simulink model "model (1)"  (R2014b)
settings: Solver=ode45  StartTime=0.0  StopTime=300  RelTol=1e-3
settings Model: Creator=User  LastModifiedBy=User

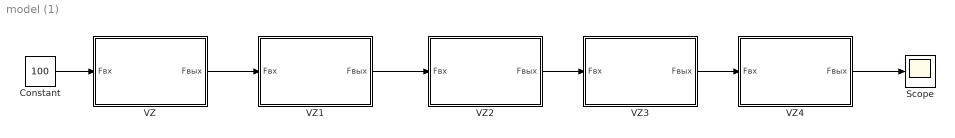
== system model (1) ==
  Constant : Constant  Value=100
  Scope : Scope
  VZ : Subsystem
  VZ1 : Subsystem
  VZ2 : Subsystem
  VZ3 : Subsystem
  VZ4 : Subsystem
  wires:
  VZ/1(Fвых) -> VZ1/1(Fвх)
  VZ4/1(Fвых) -> Scope/1
  Constant/1 -> VZ/1(Fвх)
  VZ1/1(Fвых) -> VZ2/1(Fвх)
  VZ2/1(Fвых) -> VZ3/1(Fвх)
  VZ3/1(Fвых) -> VZ4/1(Fвх)

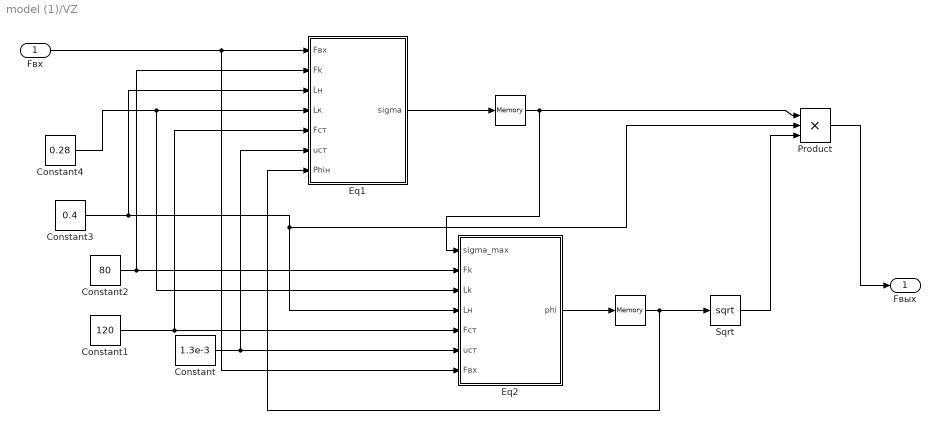
== system model (1)/VZ ==
  Fвх : Inport
  " " : Memory
  "  " : Memory
  Constant : Constant  Value=1.3e-3
  Constant1 : Constant  Value=120
  Constant2 : Constant  Value=80
  Constant3 : Constant  Value=0.4
  Constant4 : Constant  Value=0.28
  Eq1 : Subsystem  TreatAsAtomicUnit=on
  Eq2 : Subsystem  TreatAsAtomicUnit=on
  Product : Product  Inputs=3
  Sqrt : Sqrt  SaturateOnIntegerOverflow=on
  Fвых : Outport
  wires:
  Constant2/1 -> Eq2/2(Fk), Eq1/2(Fk)
  Fвх/1 -> Eq2/7(Fвх), Eq1/1(Fвх)
  Constant1/1 -> Eq1/5(Fст), Eq2/5(Fст)
  Constant4/1 -> Eq2/3(Lk), Eq1/4(Lк)
  Constant3/1 -> Eq1/3(Lн), Product/2, Eq2/4(Lн)
  Eq1/1(sigma) -> " "/1
  "  "/1 -> Eq1/7(Phiн), Sqrt/1
  " "/1 -> Product/1, Eq2/1(sigma_max)
  Eq2/1(phi) -> "  "/1
  Constant/1 -> Eq1/6(uст), Eq2/6(uст)
  Product/1 -> Fвых/1
  Sqrt/1 -> Product/3

== system model (1)/VZ1 ==
  Fвх : Inport
  " " : Memory
  "  " : Memory
  Constant : Constant  Value=1.3e-3
  Constant1 : Constant  Value=120
  Constant2 : Constant  Value=80
  Constant3 : Constant  Value=0.4
  Constant4 : Constant  Value=0.28
  Eq1 : Subsystem  TreatAsAtomicUnit=on
  Eq2 : Subsystem  TreatAsAtomicUnit=on
  Product : Product  Inputs=3
  Sqrt : Sqrt  SaturateOnIntegerOverflow=on
  Fвых : Outport
  wires:
  Constant2/1 -> Eq2/2(Fk), Eq1/2(Fk)
  Fвх/1 -> Eq2/7(Fвх), Eq1/1(Fвх)
  Constant1/1 -> Eq1/5(Fст), Eq2/5(Fст)
  Constant4/1 -> Eq2/3(Lk), Eq1/4(Lк)
  Constant3/1 -> Eq1/3(Lн), Product/2, Eq2/4(Lн)
  Eq1/1(sigma) -> " "/1
  "  "/1 -> Eq1/7(Phiн), Sqrt/1
  " "/1 -> Product/1, Eq2/1(sigma_max)
  Eq2/1(phi) -> "  "/1
  Constant/1 -> Eq1/6(uст), Eq2/6(uст)
  Product/1 -> Fвых/1
  Sqrt/1 -> Product/3

== system model (1)/VZ2 ==
  Fвх : Inport
  " " : Memory
  "  " : Memory
  Constant : Constant  Value=1.3e-3
  Constant1 : Constant  Value=120
  Constant2 : Constant  Value=80
  Constant3 : Constant  Value=0.4
  Constant4 : Constant  Value=0.28
  Eq1 : Subsystem  TreatAsAtomicUnit=on
  Eq2 : Subsystem  TreatAsAtomicUnit=on
  Product : Product  Inputs=3
  Sqrt : Sqrt  SaturateOnIntegerOverflow=on
  Fвых : Outport
  wires:
  Constant2/1 -> Eq2/2(Fk), Eq1/2(Fk)
  Fвх/1 -> Eq2/7(Fвх), Eq1/1(Fвх)
  Constant1/1 -> Eq1/5(Fст), Eq2/5(Fст)
  Constant4/1 -> Eq2/3(Lk), Eq1/4(Lк)
  Constant3/1 -> Eq1/3(Lн), Product/2, Eq2/4(Lн)
  Eq1/1(sigma) -> " "/1
  "  "/1 -> Eq1/7(Phiн), Sqrt/1
  " "/1 -> Product/1, Eq2/1(sigma_max)
  Eq2/1(phi) -> "  "/1
  Constant/1 -> Eq1/6(uст), Eq2/6(uст)
  Product/1 -> Fвых/1
  Sqrt/1 -> Product/3

== system model (1)/VZ3 ==
  Fвх : Inport
  " " : Memory
  "  " : Memory
  Constant : Constant  Value=1.3e-3
  Constant1 : Constant  Value=120
  Constant2 : Constant  Value=80
  Constant3 : Constant  Value=0.4
  Constant4 : Constant  Value=0.28
  Eq1 : Subsystem  TreatAsAtomicUnit=on
  Eq2 : Subsystem  TreatAsAtomicUnit=on
  Product : Product  Inputs=3
  Sqrt : Sqrt  SaturateOnIntegerOverflow=on
  Fвых : Outport
  wires:
  Constant2/1 -> Eq2/2(Fk), Eq1/2(Fk)
  Fвх/1 -> Eq2/7(Fвх), Eq1/1(Fвх)
  Constant1/1 -> Eq1/5(Fст), Eq2/5(Fст)
  Constant4/1 -> Eq2/3(Lk), Eq1/4(Lк)
  Constant3/1 -> Eq1/3(Lн), Product/2, Eq2/4(Lн)
  Eq1/1(sigma) -> " "/1
  "  "/1 -> Eq1/7(Phiн), Sqrt/1
  " "/1 -> Product/1, Eq2/1(sigma_max)
  Eq2/1(phi) -> "  "/1
  Constant/1 -> Eq1/6(uст), Eq2/6(uст)
  Product/1 -> Fвых/1
  Sqrt/1 -> Product/3

== system model (1)/VZ4 ==
  Fвх : Inport
  " " : Memory
  "  " : Memory
  Constant : Constant  Value=1.3e-3
  Constant1 : Constant  Value=120
  Constant2 : Constant  Value=80
  Constant3 : Constant  Value=0.4
  Constant4 : Constant  Value=0.28
  Eq1 : Subsystem  TreatAsAtomicUnit=on
  Eq2 : Subsystem  TreatAsAtomicUnit=on
  Product : Product  Inputs=3
  Sqrt : Sqrt  SaturateOnIntegerOverflow=on
  Fвых : Outport
  wires:
  Constant2/1 -> Eq2/2(Fk), Eq1/2(Fk)
  Fвх/1 -> Eq2/7(Fвх), Eq1/1(Fвх)
  Constant1/1 -> Eq1/5(Fст), Eq2/5(Fст)
  Constant4/1 -> Eq2/3(Lk), Eq1/4(Lк)
  Constant3/1 -> Eq1/3(Lн), Product/2, Eq2/4(Lн)
  Eq1/1(sigma) -> " "/1
  "  "/1 -> Eq1/7(Phiн), Sqrt/1
  " "/1 -> Product/1, Eq2/1(sigma_max)
  Eq2/1(phi) -> "  "/1
  Constant/1 -> Eq1/6(uст), Eq2/6(uст)
  Product/1 -> Fвых/1
  Sqrt/1 -> Product/3

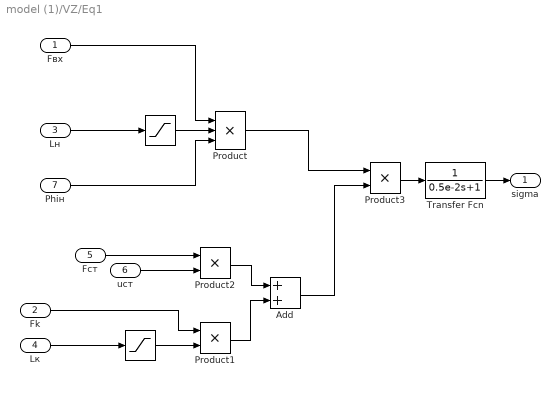
== system model (1)/VZ/Eq1 ==
  Fвх : Inport
  Fk : Inport  Port=2
  Lн : Inport  Port=3
  Lк : Inport  Port=4
  Fст : Inport  Port=5
  uст : Inport  Port=6
  Phiн : Inport  Port=7
  " " : Saturate
  "  " : Saturate
  Add : Sum
  Product : Product  Inputs=3
  Product1 : Product
  Product2 : Product
  Product3 : Product  Inputs=**
  Transfer Fcn : TransferFcn  Denominator=[0.5e-2 1]
  sigma : Outport
  wires:
  Lн/1 -> " "/1
  Lк/1 -> "  "/1
  " "/1 -> Product/2
  Fвх/1 -> Product/1
  Phiн/1 -> Product/3
  "  "/1 -> Product1/2
  Fk/1 -> Product1/1
  Fст/1 -> Product2/1
  uст/1 -> Product2/2
  Product2/1 -> Add/1
  Product1/1 -> Add/2
  Product/1 -> Product3/1
  Add/1 -> Product3/2
  Product3/1 -> Transfer Fcn/1
  Transfer Fcn/1 -> sigma/1

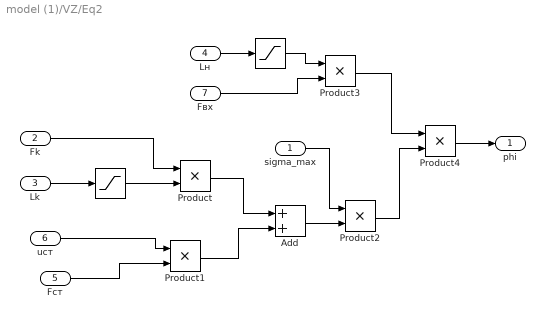
== system model (1)/VZ/Eq2 ==
  sigma_max : Inport
  Fk : Inport  Port=2
  Lk : Inport  Port=3
  Lн : Inport  Port=4
  Fст : Inport  Port=5
  uст : Inport  Port=6
  Fвх : Inport  Port=7
  " " : Saturate
  "  " : Saturate
  Add : Sum
  Product{,1..3} (4 alike) : Product
  Product4 : Product  Inputs=**
  phi : Outport
  wires:
  Lk/1 -> " "/1
  " "/1 -> Product/2
  Fk/1 -> Product/1
  uст/1 -> Product1/1
  Product/1 -> Add/1
  Product1/1 -> Add/2
  Fст/1 -> Product1/2
  Lн/1 -> "  "/1
  Add/1 -> Product2/2
  sigma_max/1 -> Product2/1
  "  "/1 -> Product3/1
  Fвх/1 -> Product3/2
  Product3/1 -> Product4/1
  Product2/1 -> Product4/2
  Product4/1 -> phi/1

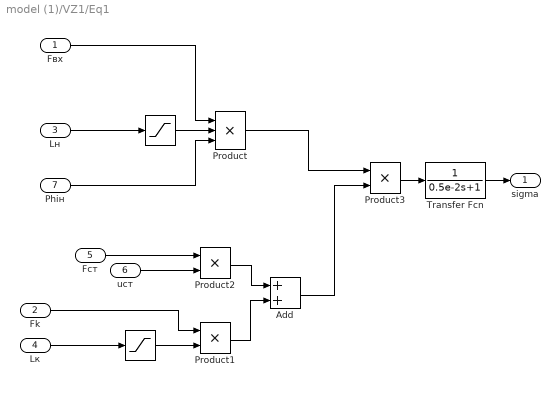
== system model (1)/VZ1/Eq1 ==
  Fвх : Inport
  Fk : Inport  Port=2
  Lн : Inport  Port=3
  Lк : Inport  Port=4
  Fст : Inport  Port=5
  uст : Inport  Port=6
  Phiн : Inport  Port=7
  " " : Saturate
  "  " : Saturate
  Add : Sum
  Product : Product  Inputs=3
  Product1 : Product
  Product2 : Product
  Product3 : Product  Inputs=**
  Transfer Fcn : TransferFcn  Denominator=[0.5e-2 1]
  sigma : Outport
  wires:
  Lн/1 -> " "/1
  Lк/1 -> "  "/1
  " "/1 -> Product/2
  Fвх/1 -> Product/1
  Phiн/1 -> Product/3
  "  "/1 -> Product1/2
  Fk/1 -> Product1/1
  Fст/1 -> Product2/1
  uст/1 -> Product2/2
  Product2/1 -> Add/1
  Product1/1 -> Add/2
  Product/1 -> Product3/1
  Add/1 -> Product3/2
  Product3/1 -> Transfer Fcn/1
  Transfer Fcn/1 -> sigma/1

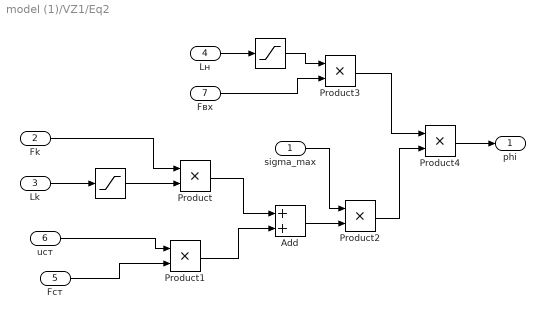
== system model (1)/VZ1/Eq2 ==
  sigma_max : Inport
  Fk : Inport  Port=2
  Lk : Inport  Port=3
  Lн : Inport  Port=4
  Fст : Inport  Port=5
  uст : Inport  Port=6
  Fвх : Inport  Port=7
  " " : Saturate
  "  " : Saturate
  Add : Sum
  Product{,1..3} (4 alike) : Product
  Product4 : Product  Inputs=**
  phi : Outport
  wires:
  Lk/1 -> " "/1
  " "/1 -> Product/2
  Fk/1 -> Product/1
  uст/1 -> Product1/1
  Product/1 -> Add/1
  Product1/1 -> Add/2
  Fст/1 -> Product1/2
  Lн/1 -> "  "/1
  Add/1 -> Product2/2
  sigma_max/1 -> Product2/1
  "  "/1 -> Product3/1
  Fвх/1 -> Product3/2
  Product3/1 -> Product4/1
  Product2/1 -> Product4/2
  Product4/1 -> phi/1

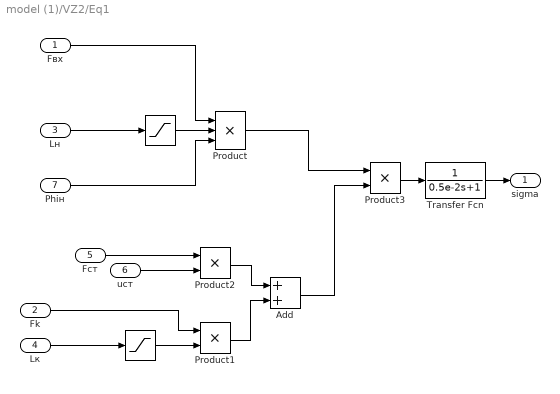
== system model (1)/VZ2/Eq1 ==
  Fвх : Inport
  Fk : Inport  Port=2
  Lн : Inport  Port=3
  Lк : Inport  Port=4
  Fст : Inport  Port=5
  uст : Inport  Port=6
  Phiн : Inport  Port=7
  " " : Saturate
  "  " : Saturate
  Add : Sum
  Product : Product  Inputs=3
  Product1 : Product
  Product2 : Product
  Product3 : Product  Inputs=**
  Transfer Fcn : TransferFcn  Denominator=[0.5e-2 1]
  sigma : Outport
  wires:
  Lн/1 -> " "/1
  Lк/1 -> "  "/1
  " "/1 -> Product/2
  Fвх/1 -> Product/1
  Phiн/1 -> Product/3
  "  "/1 -> Product1/2
  Fk/1 -> Product1/1
  Fст/1 -> Product2/1
  uст/1 -> Product2/2
  Product2/1 -> Add/1
  Product1/1 -> Add/2
  Product/1 -> Product3/1
  Add/1 -> Product3/2
  Product3/1 -> Transfer Fcn/1
  Transfer Fcn/1 -> sigma/1

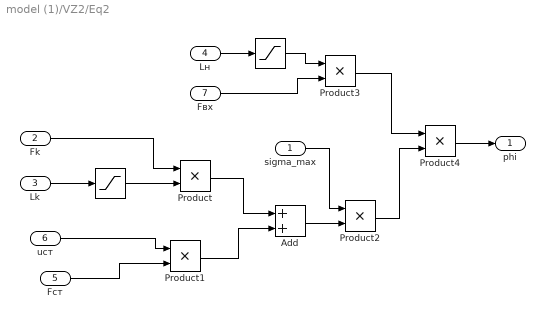
== system model (1)/VZ2/Eq2 ==
  sigma_max : Inport
  Fk : Inport  Port=2
  Lk : Inport  Port=3
  Lн : Inport  Port=4
  Fст : Inport  Port=5
  uст : Inport  Port=6
  Fвх : Inport  Port=7
  " " : Saturate
  "  " : Saturate
  Add : Sum
  Product{,1..3} (4 alike) : Product
  Product4 : Product  Inputs=**
  phi : Outport
  wires:
  Lk/1 -> " "/1
  " "/1 -> Product/2
  Fk/1 -> Product/1
  uст/1 -> Product1/1
  Product/1 -> Add/1
  Product1/1 -> Add/2
  Fст/1 -> Product1/2
  Lн/1 -> "  "/1
  Add/1 -> Product2/2
  sigma_max/1 -> Product2/1
  "  "/1 -> Product3/1
  Fвх/1 -> Product3/2
  Product3/1 -> Product4/1
  Product2/1 -> Product4/2
  Product4/1 -> phi/1

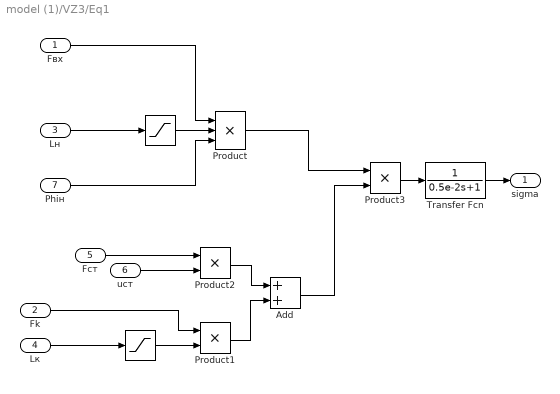
== system model (1)/VZ3/Eq1 ==
  Fвх : Inport
  Fk : Inport  Port=2
  Lн : Inport  Port=3
  Lк : Inport  Port=4
  Fст : Inport  Port=5
  uст : Inport  Port=6
  Phiн : Inport  Port=7
  " " : Saturate
  "  " : Saturate
  Add : Sum
  Product : Product  Inputs=3
  Product1 : Product
  Product2 : Product
  Product3 : Product  Inputs=**
  Transfer Fcn : TransferFcn  Denominator=[0.5e-2 1]
  sigma : Outport
  wires:
  Lн/1 -> " "/1
  Lк/1 -> "  "/1
  " "/1 -> Product/2
  Fвх/1 -> Product/1
  Phiн/1 -> Product/3
  "  "/1 -> Product1/2
  Fk/1 -> Product1/1
  Fст/1 -> Product2/1
  uст/1 -> Product2/2
  Product2/1 -> Add/1
  Product1/1 -> Add/2
  Product/1 -> Product3/1
  Add/1 -> Product3/2
  Product3/1 -> Transfer Fcn/1
  Transfer Fcn/1 -> sigma/1

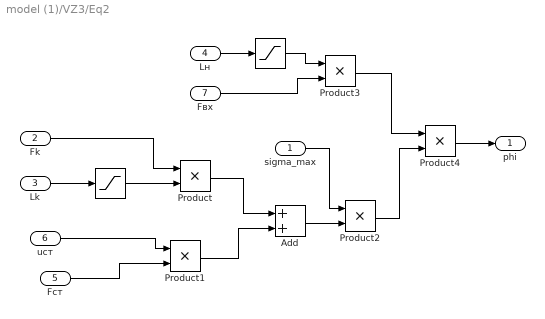
== system model (1)/VZ3/Eq2 ==
  sigma_max : Inport
  Fk : Inport  Port=2
  Lk : Inport  Port=3
  Lн : Inport  Port=4
  Fст : Inport  Port=5
  uст : Inport  Port=6
  Fвх : Inport  Port=7
  " " : Saturate
  "  " : Saturate
  Add : Sum
  Product{,1..3} (4 alike) : Product
  Product4 : Product  Inputs=**
  phi : Outport
  wires:
  Lk/1 -> " "/1
  " "/1 -> Product/2
  Fk/1 -> Product/1
  uст/1 -> Product1/1
  Product/1 -> Add/1
  Product1/1 -> Add/2
  Fст/1 -> Product1/2
  Lн/1 -> "  "/1
  Add/1 -> Product2/2
  sigma_max/1 -> Product2/1
  "  "/1 -> Product3/1
  Fвх/1 -> Product3/2
  Product3/1 -> Product4/1
  Product2/1 -> Product4/2
  Product4/1 -> phi/1

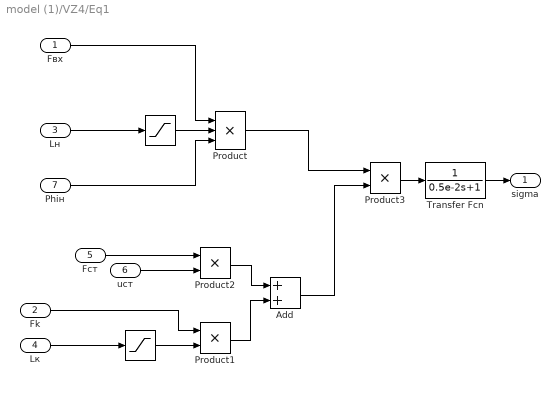
== system model (1)/VZ4/Eq1 ==
  Fвх : Inport
  Fk : Inport  Port=2
  Lн : Inport  Port=3
  Lк : Inport  Port=4
  Fст : Inport  Port=5
  uст : Inport  Port=6
  Phiн : Inport  Port=7
  " " : Saturate
  "  " : Saturate
  Add : Sum
  Product : Product  Inputs=3
  Product1 : Product
  Product2 : Product
  Product3 : Product  Inputs=**
  Transfer Fcn : TransferFcn  Denominator=[0.5e-2 1]
  sigma : Outport
  wires:
  Lн/1 -> " "/1
  Lк/1 -> "  "/1
  " "/1 -> Product/2
  Fвх/1 -> Product/1
  Phiн/1 -> Product/3
  "  "/1 -> Product1/2
  Fk/1 -> Product1/1
  Fст/1 -> Product2/1
  uст/1 -> Product2/2
  Product2/1 -> Add/1
  Product1/1 -> Add/2
  Product/1 -> Product3/1
  Add/1 -> Product3/2
  Product3/1 -> Transfer Fcn/1
  Transfer Fcn/1 -> sigma/1

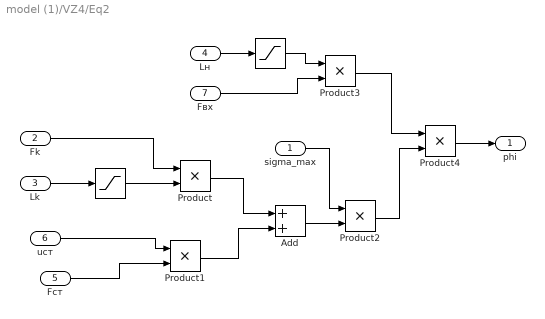
== system model (1)/VZ4/Eq2 ==
  sigma_max : Inport
  Fk : Inport  Port=2
  Lk : Inport  Port=3
  Lн : Inport  Port=4
  Fст : Inport  Port=5
  uст : Inport  Port=6
  Fвх : Inport  Port=7
  " " : Saturate
  "  " : Saturate
  Add : Sum
  Product{,1..3} (4 alike) : Product
  Product4 : Product  Inputs=**
  phi : Outport
  wires:
  Lk/1 -> " "/1
  " "/1 -> Product/2
  Fk/1 -> Product/1
  uст/1 -> Product1/1
  Product/1 -> Add/1
  Product1/1 -> Add/2
  Fст/1 -> Product1/2
  Lн/1 -> "  "/1
  Add/1 -> Product2/2
  sigma_max/1 -> Product2/1
  "  "/1 -> Product3/1
  Fвх/1 -> Product3/2
  Product3/1 -> Product4/1
  Product2/1 -> Product4/2
  Product4/1 -> phi/1
